simulink model "doublemass"  (R2022b)
settings: Solver=FixedStepAuto  StartTime=0.0  StopTime=10.0  FixedStep=0.02  RelTol=1e-3
model workspace (MAT data in the model file):
  a_max = 10
  a_min = -10
  adva_max = [0.001 0.001 0.001 0.001]
  adva_min = [-0.001 -0.001 -0.001 -0.001]
  ka = 50
  m1 = 10
  m2 = 10
  x_ini = Simulink.Parameter
  x_ini.Value = [-0.1 0 0.1 0]
  x_ini.DataType = 'auto'
  x_ini.Complexity = 'real'
  x_ini.Dimensions = [1 4]
libraries: simulink x1
settings Model: TunableVars=a_max,a_min,adva_max,adva_min,x_ini,x_max,x_min  TunableVarsStorageClass=Auto,Auto,Auto,Auto,Auto,Auto,Auto  TunableVarsTypeQualifier=,,,,,,  ParameterArgumentNames=x_ini  Creator=hjzsj  LastModifiedBy=Yuxuan
settings ConfigSet: Description=Config for code generation python binding.
settings SolverCC: AlgebraicLoopSolver=TrustRegion
settings OptimizationCC: DefaultParameterBehavior=Inlined  UseDivisionForNetSlopeComputation=on  UseFloatMulNetSlope=on  StrengthReduction=on  PassReuseOutputArgsAs=Individual arguments  ZeroExternalMemoryAtStartup=off  ZeroInternalMemoryAtStartup=off  NoFixptDivByZeroProtection=on  EfficientFloat2IntCast=on  OptimizeBlockOrder=speed  OptimizationPriority=Speed  OptimizationCustomize=off  MultiThreadedLoops=on  EfficientTunableParamExpr=on
settings DebuggingCC: ParameterTunabilityLossMsg=error  UnconnectedInputMsg=warning  UnconnectedOutputMsg=warning  UnconnectedLineMsg=warning  SFMachineParentedDataDiag=warning  ArithmeticOperatorsInVariantConditions=warning
settings HardwareCC: ProdLongLongMode=on  TargetPreprocMaxBitsSint=64  TargetPreprocMaxBitsUint=64
settings ModelReferenceCC: EnableRefExpFcnMdlSchedulingChecks=on
settings SFSimCC: MATLABDynamicMemAlloc=off  CustomCodeUndefinedFunction=UseInterfaceOnly  SimTargetLang=C++
settings RTWCC: Description=Embedded Coder  SystemTargetFile=ert.tlc  GenCodeOnly=on  TemplateMakefile=ert_default_tmf  PostCodeGenCommand=slxpy.postprocess(modelName,buildInfo)  RetainRTWFile=on  PortableWordSizes=on  TargetLang=C++
settings CodeAppCC: ForceParamTrailComments=on  CommentStyle=Multi-line  IgnoreCustomStorageClasses=off  MaxIdLength=64  OperatorAnnotations=on  SimulinkDataObjDesc=on  SFDataObjDesc=on  MATLABFcnDesc=on  MangleLength=4  InsertBlockDesc=on  StateflowObjectComments=on  MATLABSourceComments=on
settings ERTTargetCC: TargetLangStandard=C++11 (ISO)  SupportAbsoluteTime=off  CodeInterfacePackaging=C++ class  SupportNonFinite=off  SupportComplex=off  SupportContinuousTime=on  InlinedParameterPlacement=NonHierarchical  RootIOFormat=Structure reference  ERTCustomFileTemplate=example_file_process.tlc

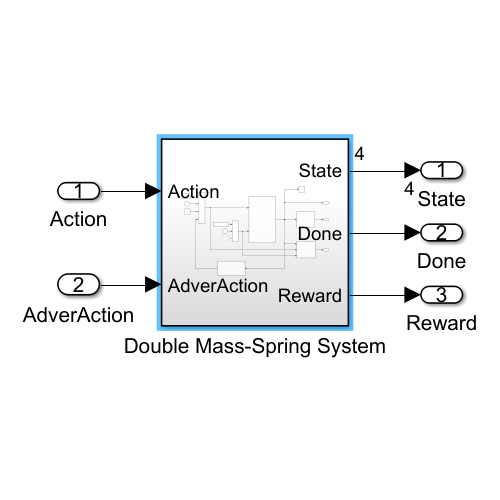
[thumbnail: Simulink's stored preview of the top-level diagram]
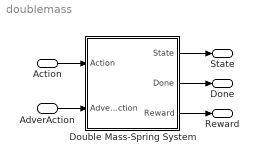
== system doublemass ==
  Action : Inport
  AdverAction : Inport  Port=2
  Double Mass-Spring System : Subsystem
  State : Outport
  Done : Outport  Port=2
  Reward : Outport  Port=3
  wires:
  Double Mass-Spring System/1(State) -> State/1
  Double Mass-Spring System/2(Done) -> Done/1
  Action/1 -> Double Mass-Spring System/1(Action)
  Double Mass-Spring System/3(Reward) -> Reward/1
  AdverAction/1 -> Double Mass-Spring System/2(AdverAction)

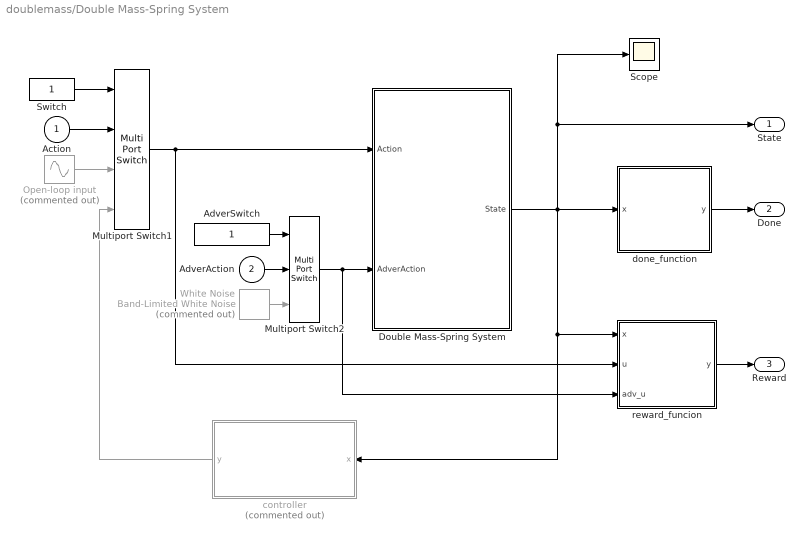
== system doublemass/Double Mass-Spring System ==
  Action : Inport
  AdverAction : Inport  Port=2
  AdverSwitch : Constant
  Double Mass-Spring System : Subsystem
  Multiport Switch1 : MultiPortSwitch  SaturateOnIntegerOverflow=off  InputSameDT=off
  Multiport Switch2 : MultiPortSwitch  Inputs=2  SaturateOnIntegerOverflow=off  InputSameDT=off
  Open-loop input : Sin  Commented=on  SampleTime=0
  Scope : Scope
  Switch : Constant
  White Noise : simulink/Sources/Band-Limited White Noise  Commented=on  Cov=[0.5]  Ts=0.02  seed=[23341]
  controller : MATLAB Function  Commented=on  TreatAsAtomicUnit=on
  done_function : MATLAB Function  TreatAsAtomicUnit=on
  reward_funcion : MATLAB Function  TreatAsAtomicUnit=on
  State : Outport
  Done : Outport  Port=2
  Reward : Outport  Port=3
  wires:
  done_function/1(y) -> Done/1
  reward_funcion/1(y) -> Reward/1
  controller/1(y) -> Multiport Switch1/4
  Switch/1 -> Multiport Switch1/1
  Action/1 -> Multiport Switch1/2
  Double Mass-Spring System/1(State) -> controller/1(x), reward_funcion/1(x), done_function/1(x), Scope/1, State/1
  Multiport Switch1/1 -> reward_funcion/2(u), Double Mass-Spring System/1(Action)
  Open-loop input/1 -> Multiport Switch1/3
  Multiport Switch2/1 -> reward_funcion/3(adv_u), Double Mass-Spring System/2(AdverAction)
  AdverSwitch/1 -> Multiport Switch2/1
  White Noise/1 -> Multiport Switch2/3
  AdverAction/1 -> Multiport Switch2/2

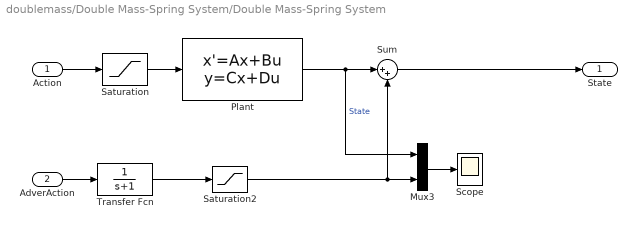
== system doublemass/Double Mass-Spring System/Double Mass-Spring System ==
  Action : Inport
  AdverAction : Inport  Port=2
  Mux3 : Mux  Inputs=2
  Plant : StateSpace  A=[0 1 0 0; -ka/m1 0 ka/m1 0; 0 0 0 1;ka/m2 0 -ka/m2 0]  B=[0; 1; 0; 0]  C=[1 0 0 0;0 1 0 0;0 0 1 0;0 0 0 1]  D=zeros(4,1)  InitialCondition=x_ini
  Saturation : Saturate  UpperLimit=a_max  LowerLimit=a_min
  Saturation2 : Saturate  UpperLimit=adva_max  LowerLimit=adva_min
  Scope : Scope
  Sum : Sum  Inputs=|++
  Transfer Fcn : TransferFcn  Denominator=[1 1]
  State : Outport
  wires:
  Saturation/1 -> Plant/1
  Action/1 -> Saturation/1
  Sum/1 -> State/1
  Transfer Fcn/1 -> Saturation2/1
  Mux3/1 -> Scope/1
  AdverAction/1 -> Transfer Fcn/1
  Saturation2/1 -> Sum/2, Mux3/2
  Plant/1 -> Mux3/1, Sum/1  "State"

== matlab function doublemass/Double Mass-Spring System/controller ==
  data: x input size=4; y output
function y = fcn(x)
done = (abs(x(1)) > 2.4)||(abs(x(3)) > 0.2094);
y = done;

== matlab function doublemass/Double Mass-Spring System/done_function ==
  data: x input; y output
function y = fcn(x)
done = (  (abs(x(3))>5) || ((abs(x(3)-0)<0.01) && (abs(x(4))<0.01)) || (x(3)>x(1))  );
y = done;

== matlab function doublemass/Double Mass-Spring System/reward_funcion ==
  data: x input; y output; u input; adv_u input
function y = fcn(x, u, adv_u)
reward = -(x(3)-0)^2-5*(x(4)-0)^2-0.2*u^2;
y = reward;
